simulink model "NPC_grid_tied"  (R2020a)
settings: Solver=ode8  StartTime=0.0  StopTime=0.1  FixedStep=1e-6  RelTol=1e-3
libraries: powerlib x31, simulink x6
(part 2 of 2)

== system NPC_grid_tied/SVPWM/state/2/Subsystem6 ==
  M : Inport
  Constant : Constant  Value=[0 1 0]
  Constant1 : Constant  Value=[1 1 0]
  Constant2 : Constant  Value=[1 1 1]
  Constant3 : Constant  Value=[1 2 1]
  Constant4 : Constant  Value=[1 1 0]
  Constant5 : Constant  Value=[1 1 1]
  Constant6 : Constant  Value=[0 1 0]
  Multiport Switch : MultiPortSwitch  Inputs=7
  state : Outport  VectorParamsAs1DForOutWhenUnconnected=off
  wires:
  Multiport Switch/1 -> state/1
  M/1 -> Multiport Switch/1
  Constant/1 -> Multiport Switch/2
  Constant1/1 -> Multiport Switch/3
  Constant2/1 -> Multiport Switch/4
  Constant3/1 -> Multiport Switch/5
  Constant5/1 -> Multiport Switch/6
  Constant4/1 -> Multiport Switch/7
  Constant6/1 -> Multiport Switch/8

== system NPC_grid_tied/SVPWM/state/2/Subsystem7 ==
  M : Inport
  Constant : Constant  Value=[1 1 0]
  Constant1 : Constant  Value=[1 2 0]
  Constant2 : Constant  Value=[1 2 1]
  Constant3 : Constant  Value=[2 2 1]
  Constant4 : Constant  Value=[1 2 0]
  Constant5 : Constant  Value=[1 2 1]
  Constant6 : Constant  Value=[1 1 0]
  Multiport Switch : MultiPortSwitch  Inputs=7
  state : Outport  VectorParamsAs1DForOutWhenUnconnected=off
  wires:
  Constant6/1 -> Multiport Switch/8
  Constant4/1 -> Multiport Switch/7
  Constant5/1 -> Multiport Switch/6
  Constant3/1 -> Multiport Switch/5
  Constant2/1 -> Multiport Switch/4
  Constant1/1 -> Multiport Switch/3
  Constant/1 -> Multiport Switch/2
  M/1 -> Multiport Switch/1
  Multiport Switch/1 -> state/1

== system NPC_grid_tied/SVPWM/state/2/Subsystem8 ==
  M : Inport
  Constant : Constant  Value=[0 1 0]
  Constant1 : Constant  Value=[1 1 0]
  Constant2 : Constant  Value=[1 2 0]
  Constant3 : Constant  Value=[1 2 1]
  Constant4 : Constant  Value=[1 1 0]
  Constant5 : Constant  Value=[1 2 0]
  Constant6 : Constant  Value=[0 1 0]
  Multiport Switch : MultiPortSwitch  Inputs=7
  state : Outport  VectorParamsAs1DForOutWhenUnconnected=off
  wires:
  Multiport Switch/1 -> state/1
  M/1 -> Multiport Switch/1
  Constant/1 -> Multiport Switch/2
  Constant1/1 -> Multiport Switch/3
  Constant2/1 -> Multiport Switch/4
  Constant3/1 -> Multiport Switch/5
  Constant5/1 -> Multiport Switch/6
  Constant4/1 -> Multiport Switch/7
  Constant6/1 -> Multiport Switch/8

== system NPC_grid_tied/SVPWM/state/2/Subsystem9 ==
  M : Inport
  Constant : Constant  Value=[1 1 0]
  Constant1 : Constant  Value=[1 2 0]
  Constant2 : Constant  Value=[2 2 0]
  Constant3 : Constant  Value=[2 2 1]
  Constant4 : Constant  Value=[1 2 0]
  Constant5 : Constant  Value=[2 2 0]
  Constant6 : Constant  Value=[1 1 0]
  Multiport Switch : MultiPortSwitch  Inputs=7
  state : Outport  VectorParamsAs1DForOutWhenUnconnected=off
  wires:
  Constant6/1 -> Multiport Switch/8
  Constant4/1 -> Multiport Switch/7
  Constant5/1 -> Multiport Switch/6
  Constant3/1 -> Multiport Switch/5
  Constant2/1 -> Multiport Switch/4
  Constant1/1 -> Multiport Switch/3
  Constant/1 -> Multiport Switch/2
  M/1 -> Multiport Switch/1
  Multiport Switch/1 -> state/1

== system NPC_grid_tied/SVPWM/state/3/Subsystem10 ==
  M : Inport
  Constant : Constant  Value=[0 1 1]
  Constant1 : Constant  Value=[0 2 1]
  Constant2 : Constant  Value=[0 2 2]
  Constant3 : Constant  Value=[1 2 2]
  Constant4 : Constant  Value=[0 2 1]
  Constant5 : Constant  Value=[0 2 2]
  Constant6 : Constant  Value=[0 1 1]
  Multiport Switch : MultiPortSwitch  Inputs=7
  state : Outport  VectorParamsAs1DForOutWhenUnconnected=off
  wires:
  Constant6/1 -> Multiport Switch/8
  Constant4/1 -> Multiport Switch/7
  Constant5/1 -> Multiport Switch/6
  Constant3/1 -> Multiport Switch/5
  Constant2/1 -> Multiport Switch/4
  Constant1/1 -> Multiport Switch/3
  Constant/1 -> Multiport Switch/2
  M/1 -> Multiport Switch/1
  Multiport Switch/1 -> state/1

== system NPC_grid_tied/SVPWM/state/3/Subsystem5 ==
  M : Inport
  Constant : Constant  Value=[0 1 0]
  Constant1 : Constant  Value=[0 1 1]
  Constant2 : Constant  Value=[1 1 1]
  Constant3 : Constant  Value=[1 2 1]
  Constant4 : Constant  Value=[0 1 1]
  Constant5 : Constant  Value=[1 1 1]
  Constant6 : Constant  Value=[0 1 0]
  Multiport Switch : MultiPortSwitch  Inputs=7
  state : Outport  VectorParamsAs1DForOutWhenUnconnected=off
  wires:
  Multiport Switch/1 -> state/1
  M/1 -> Multiport Switch/1
  Constant/1 -> Multiport Switch/2
  Constant1/1 -> Multiport Switch/3
  Constant2/1 -> Multiport Switch/4
  Constant3/1 -> Multiport Switch/5
  Constant5/1 -> Multiport Switch/6
  Constant4/1 -> Multiport Switch/7
  Constant6/1 -> Multiport Switch/8

== system NPC_grid_tied/SVPWM/state/3/Subsystem6 ==
  M : Inport
  Constant : Constant  Value=[0 1 1]
  Constant1 : Constant  Value=[1 1 1]
  Constant2 : Constant  Value=[1 2 1]
  Constant3 : Constant  Value=[1 2 2]
  Constant4 : Constant  Value=[1 1 1]
  Constant5 : Constant  Value=[1 2 1]
  Constant6 : Constant  Value=[0 1 1]
  Multiport Switch : MultiPortSwitch  Inputs=7
  state : Outport  VectorParamsAs1DForOutWhenUnconnected=off
  wires:
  Constant6/1 -> Multiport Switch/8
  Constant4/1 -> Multiport Switch/7
  Constant5/1 -> Multiport Switch/6
  Constant3/1 -> Multiport Switch/5
  Constant2/1 -> Multiport Switch/4
  Constant1/1 -> Multiport Switch/3
  Constant/1 -> Multiport Switch/2
  M/1 -> Multiport Switch/1
  Multiport Switch/1 -> state/1

== system NPC_grid_tied/SVPWM/state/3/Subsystem7 ==
  M : Inport
  Constant : Constant  Value=[0 1 0]
  Constant1 : Constant  Value=[0 1 1]
  Constant2 : Constant  Value=[0 2 1]
  Constant3 : Constant  Value=[1 2 1]
  Constant4 : Constant  Value=[0 1 1]
  Constant5 : Constant  Value=[0 2 1]
  Constant6 : Constant  Value=[0 1 0]
  Multiport Switch : MultiPortSwitch  Inputs=7
  state : Outport  VectorParamsAs1DForOutWhenUnconnected=off
  wires:
  Multiport Switch/1 -> state/1
  M/1 -> Multiport Switch/1
  Constant/1 -> Multiport Switch/2
  Constant1/1 -> Multiport Switch/3
  Constant2/1 -> Multiport Switch/4
  Constant3/1 -> Multiport Switch/5
  Constant5/1 -> Multiport Switch/6
  Constant4/1 -> Multiport Switch/7
  Constant6/1 -> Multiport Switch/8

== system NPC_grid_tied/SVPWM/state/3/Subsystem8 ==
  M : Inport
  Constant : Constant  Value=[0 1 1]
  Constant1 : Constant  Value=[0 2 1]
  Constant2 : Constant  Value=[1 2 1]
  Constant3 : Constant  Value=[1 2 2]
  Constant4 : Constant  Value=[0 2 1]
  Constant5 : Constant  Value=[1 2 1]
  Constant6 : Constant  Value=[0 1 1]
  Multiport Switch : MultiPortSwitch  Inputs=7
  state : Outport  VectorParamsAs1DForOutWhenUnconnected=off
  wires:
  Constant6/1 -> Multiport Switch/8
  Constant4/1 -> Multiport Switch/7
  Constant5/1 -> Multiport Switch/6
  Constant3/1 -> Multiport Switch/5
  Constant2/1 -> Multiport Switch/4
  Constant1/1 -> Multiport Switch/3
  Constant/1 -> Multiport Switch/2
  M/1 -> Multiport Switch/1
  Multiport Switch/1 -> state/1

== system NPC_grid_tied/SVPWM/state/3/Subsystem9 ==
  M : Inport
  Constant : Constant  Value=[0 1 0]
  Constant1 : Constant  Value=[0 2 0]
  Constant2 : Constant  Value=[0 2 1]
  Constant3 : Constant  Value=[1 2 1]
  Constant4 : Constant  Value=[0 2 0]
  Constant5 : Constant  Value=[0 2 1]
  Constant6 : Constant  Value=[0 1 0]
  Multiport Switch : MultiPortSwitch  Inputs=7
  state : Outport  VectorParamsAs1DForOutWhenUnconnected=off
  wires:
  Multiport Switch/1 -> state/1
  M/1 -> Multiport Switch/1
  Constant/1 -> Multiport Switch/2
  Constant1/1 -> Multiport Switch/3
  Constant2/1 -> Multiport Switch/4
  Constant3/1 -> Multiport Switch/5
  Constant5/1 -> Multiport Switch/6
  Constant4/1 -> Multiport Switch/7
  Constant6/1 -> Multiport Switch/8

== system NPC_grid_tied/SVPWM/state/4/Subsystem10 ==
  M : Inport
  Constant : Constant  Value=[0 0 1]
  Constant1 : Constant  Value=[0 0 2]
  Constant2 : Constant  Value=[0 1 2]
  Constant3 : Constant  Value=[1 1 2]
  Constant4 : Constant  Value=[0 0 2]
  Constant5 : Constant  Value=[0 1 2]
  Constant6 : Constant  Value=[0 0 1]
  Multiport Switch : MultiPortSwitch  Inputs=7
  state : Outport  VectorParamsAs1DForOutWhenUnconnected=off
  wires:
  Multiport Switch/1 -> state/1
  M/1 -> Multiport Switch/1
  Constant/1 -> Multiport Switch/2
  Constant1/1 -> Multiport Switch/3
  Constant2/1 -> Multiport Switch/4
  Constant3/1 -> Multiport Switch/5
  Constant5/1 -> Multiport Switch/6
  Constant4/1 -> Multiport Switch/7
  Constant6/1 -> Multiport Switch/8

== system NPC_grid_tied/SVPWM/state/4/Subsystem5 ==
  M : Inport
  Constant : Constant  Value=[0 1 1]
  Constant1 : Constant  Value=[1 1 1]
  Constant2 : Constant  Value=[1 1 2]
  Constant3 : Constant  Value=[1 2 2]
  Constant4 : Constant  Value=[1 1 1]
  Constant5 : Constant  Value=[1 1 2]
  Constant6 : Constant  Value=[0 1 1]
  Multiport Switch : MultiPortSwitch  Inputs=7
  state : Outport  VectorParamsAs1DForOutWhenUnconnected=off
  wires:
  Constant6/1 -> Multiport Switch/8
  Constant4/1 -> Multiport Switch/7
  Constant5/1 -> Multiport Switch/6
  Constant3/1 -> Multiport Switch/5
  Constant2/1 -> Multiport Switch/4
  Constant1/1 -> Multiport Switch/3
  Constant/1 -> Multiport Switch/2
  M/1 -> Multiport Switch/1
  Multiport Switch/1 -> state/1

== system NPC_grid_tied/SVPWM/state/4/Subsystem6 ==
  M : Inport
  Constant : Constant  Value=[0 0 1]
  Constant1 : Constant  Value=[0 1 1]
  Constant2 : Constant  Value=[1 1 1]
  Constant3 : Constant  Value=[1 1 2]
  Constant4 : Constant  Value=[0 1 1]
  Constant5 : Constant  Value=[1 1 1]
  Constant6 : Constant  Value=[0 0 1]
  Multiport Switch : MultiPortSwitch  Inputs=7
  state : Outport  VectorParamsAs1DForOutWhenUnconnected=off
  wires:
  Multiport Switch/1 -> state/1
  M/1 -> Multiport Switch/1
  Constant/1 -> Multiport Switch/2
  Constant1/1 -> Multiport Switch/3
  Constant2/1 -> Multiport Switch/4
  Constant3/1 -> Multiport Switch/5
  Constant5/1 -> Multiport Switch/6
  Constant4/1 -> Multiport Switch/7
  Constant6/1 -> Multiport Switch/8

== system NPC_grid_tied/SVPWM/state/4/Subsystem7 ==
  M : Inport
  Constant : Constant  Value=[0 1 1]
  Constant1 : Constant  Value=[0 1 2]
  Constant2 : Constant  Value=[1 1 2]
  Constant3 : Constant  Value=[1 2 2]
  Constant4 : Constant  Value=[0 1 2]
  Constant5 : Constant  Value=[1 1 2]
  Constant6 : Constant  Value=[0 1 1]
  Multiport Switch : MultiPortSwitch  Inputs=7
  state : Outport  VectorParamsAs1DForOutWhenUnconnected=off
  wires:
  Constant6/1 -> Multiport Switch/8
  Constant4/1 -> Multiport Switch/7
  Constant5/1 -> Multiport Switch/6
  Constant3/1 -> Multiport Switch/5
  Constant2/1 -> Multiport Switch/4
  Constant1/1 -> Multiport Switch/3
  Constant/1 -> Multiport Switch/2
  M/1 -> Multiport Switch/1
  Multiport Switch/1 -> state/1

== system NPC_grid_tied/SVPWM/state/4/Subsystem8 ==
  M : Inport
  Constant : Constant  Value=[0 0 1]
  Constant1 : Constant  Value=[0 1 1]
  Constant2 : Constant  Value=[0 1 2]
  Constant3 : Constant  Value=[1 1 2]
  Constant4 : Constant  Value=[0 1 1]
  Constant5 : Constant  Value=[0 1 2]
  Constant6 : Constant  Value=[0 0 1]
  Multiport Switch : MultiPortSwitch  Inputs=7
  state : Outport  VectorParamsAs1DForOutWhenUnconnected=off
  wires:
  Multiport Switch/1 -> state/1
  M/1 -> Multiport Switch/1
  Constant/1 -> Multiport Switch/2
  Constant1/1 -> Multiport Switch/3
  Constant2/1 -> Multiport Switch/4
  Constant3/1 -> Multiport Switch/5
  Constant5/1 -> Multiport Switch/6
  Constant4/1 -> Multiport Switch/7
  Constant6/1 -> Multiport Switch/8

== system NPC_grid_tied/SVPWM/state/4/Subsystem9 ==
  M : Inport
  Constant : Constant  Value=[0 1 1]
  Constant1 : Constant  Value=[0 1 2]
  Constant2 : Constant  Value=[0 2 2]
  Constant3 : Constant  Value=[1 2 2]
  Constant4 : Constant  Value=[0 1 2]
  Constant5 : Constant  Value=[0 2 2]
  Constant6 : Constant  Value=[0 1 1]
  Multiport Switch : MultiPortSwitch  Inputs=7
  state : Outport  VectorParamsAs1DForOutWhenUnconnected=off
  wires:
  Constant6/1 -> Multiport Switch/8
  Constant4/1 -> Multiport Switch/7
  Constant5/1 -> Multiport Switch/6
  Constant3/1 -> Multiport Switch/5
  Constant2/1 -> Multiport Switch/4
  Constant1/1 -> Multiport Switch/3
  Constant/1 -> Multiport Switch/2
  M/1 -> Multiport Switch/1
  Multiport Switch/1 -> state/1

== system NPC_grid_tied/SVPWM/state/5/Subsystem10 ==
  M : Inport
  Constant : Constant  Value=[1 0 1]
  Constant1 : Constant  Value=[1 0 2]
  Constant2 : Constant  Value=[2 0 2]
  Constant3 : Constant  Value=[2 1 2]
  Constant4 : Constant  Value=[1 0 2]
  Constant5 : Constant  Value=[2 0 2]
  Constant6 : Constant  Value=[1 0 1]
  Multiport Switch : MultiPortSwitch  Inputs=7
  state : Outport  VectorParamsAs1DForOutWhenUnconnected=off
  wires:
  Constant6/1 -> Multiport Switch/8
  Constant4/1 -> Multiport Switch/7
  Constant5/1 -> Multiport Switch/6
  Constant3/1 -> Multiport Switch/5
  Constant2/1 -> Multiport Switch/4
  Constant1/1 -> Multiport Switch/3
  Constant/1 -> Multiport Switch/2
  M/1 -> Multiport Switch/1
  Multiport Switch/1 -> state/1

== system NPC_grid_tied/SVPWM/state/5/Subsystem5 ==
  M : Inport
  Constant : Constant  Value=[0 0 1]
  Constant1 : Constant  Value=[1 0 1]
  Constant2 : Constant  Value=[1 1 1]
  Constant3 : Constant  Value=[1 1 2]
  Constant4 : Constant  Value=[1 0 1]
  Constant5 : Constant  Value=[1 1 1]
  Constant6 : Constant  Value=[0 0 1]
  Multiport Switch : MultiPortSwitch  Inputs=7
  state : Outport  VectorParamsAs1DForOutWhenUnconnected=off
  wires:
  Multiport Switch/1 -> state/1
  M/1 -> Multiport Switch/1
  Constant/1 -> Multiport Switch/2
  Constant1/1 -> Multiport Switch/3
  Constant2/1 -> Multiport Switch/4
  Constant3/1 -> Multiport Switch/5
  Constant5/1 -> Multiport Switch/6
  Constant4/1 -> Multiport Switch/7
  Constant6/1 -> Multiport Switch/8

== system NPC_grid_tied/SVPWM/state/5/Subsystem6 ==
  M : Inport
  Constant : Constant  Value=[1 0 1]
  Constant1 : Constant  Value=[1 1 1]
  Constant2 : Constant  Value=[1 1 2]
  Constant3 : Constant  Value=[2 1 2]
  Constant4 : Constant  Value=[1 1 1]
  Constant5 : Constant  Value=[1 1 2]
  Constant6 : Constant  Value=[1 0 1]
  Multiport Switch : MultiPortSwitch  Inputs=7
  state : Outport  VectorParamsAs1DForOutWhenUnconnected=off
  wires:
  Constant6/1 -> Multiport Switch/8
  Constant4/1 -> Multiport Switch/7
  Constant5/1 -> Multiport Switch/6
  Constant3/1 -> Multiport Switch/5
  Constant2/1 -> Multiport Switch/4
  Constant1/1 -> Multiport Switch/3
  Constant/1 -> Multiport Switch/2
  M/1 -> Multiport Switch/1
  Multiport Switch/1 -> state/1

== system NPC_grid_tied/SVPWM/state/5/Subsystem7 ==
  M : Inport
  Constant : Constant  Value=[0 0 1]
  Constant1 : Constant  Value=[1 0 1]
  Constant2 : Constant  Value=[1 0 2]
  Constant3 : Constant  Value=[1 1 2]
  Constant4 : Constant  Value=[1 0 1]
  Constant5 : Constant  Value=[1 0 2]
  Constant6 : Constant  Value=[0 0 1]
  Multiport Switch : MultiPortSwitch  Inputs=7
  state : Outport  VectorParamsAs1DForOutWhenUnconnected=off
  wires:
  Multiport Switch/1 -> state/1
  M/1 -> Multiport Switch/1
  Constant/1 -> Multiport Switch/2
  Constant1/1 -> Multiport Switch/3
  Constant2/1 -> Multiport Switch/4
  Constant3/1 -> Multiport Switch/5
  Constant5/1 -> Multiport Switch/6
  Constant4/1 -> Multiport Switch/7
  Constant6/1 -> Multiport Switch/8

== system NPC_grid_tied/SVPWM/state/5/Subsystem8 ==
  M : Inport
  Constant : Constant  Value=[1 0 1]
  Constant1 : Constant  Value=[1 0 2]
  Constant2 : Constant  Value=[1 1 2]
  Constant3 : Constant  Value=[2 1 2]
  Constant4 : Constant  Value=[1 0 2]
  Constant5 : Constant  Value=[1 1 2]
  Constant6 : Constant  Value=[1 0 1]
  Multiport Switch : MultiPortSwitch  Inputs=7
  state : Outport  VectorParamsAs1DForOutWhenUnconnected=off
  wires:
  Constant6/1 -> Multiport Switch/8
  Constant4/1 -> Multiport Switch/7
  Constant5/1 -> Multiport Switch/6
  Constant3/1 -> Multiport Switch/5
  Constant2/1 -> Multiport Switch/4
  Constant1/1 -> Multiport Switch/3
  Constant/1 -> Multiport Switch/2
  M/1 -> Multiport Switch/1
  Multiport Switch/1 -> state/1

== system NPC_grid_tied/SVPWM/state/5/Subsystem9 ==
  M : Inport
  Constant : Constant  Value=[0 0 1]
  Constant1 : Constant  Value=[0 0 2]
  Constant2 : Constant  Value=[1 0 2]
  Constant3 : Constant  Value=[1 1 2]
  Constant4 : Constant  Value=[0 0 2]
  Constant5 : Constant  Value=[1 0 2]
  Constant6 : Constant  Value=[0 0 1]
  Multiport Switch : MultiPortSwitch  Inputs=7
  state : Outport  VectorParamsAs1DForOutWhenUnconnected=off
  wires:
  Multiport Switch/1 -> state/1
  M/1 -> Multiport Switch/1
  Constant/1 -> Multiport Switch/2
  Constant1/1 -> Multiport Switch/3
  Constant2/1 -> Multiport Switch/4
  Constant3/1 -> Multiport Switch/5
  Constant5/1 -> Multiport Switch/6
  Constant4/1 -> Multiport Switch/7
  Constant6/1 -> Multiport Switch/8

== system NPC_grid_tied/SVPWM/state/6/Subsystem10 ==
  M : Inport
  Constant : Constant  Value=[1 0 0]
  Constant1 : Constant  Value=[2 0 0]
  Constant2 : Constant  Value=[2 0 1]
  Constant3 : Constant  Value=[2 1 1]
  Constant4 : Constant  Value=[2 0 0]
  Constant5 : Constant  Value=[2 0 1]
  Constant6 : Constant  Value=[1 0 0]
  Multiport Switch : MultiPortSwitch  Inputs=7
  state : Outport  VectorParamsAs1DForOutWhenUnconnected=off
  wires:
  Multiport Switch/1 -> state/1
  M/1 -> Multiport Switch/1
  Constant/1 -> Multiport Switch/2
  Constant1/1 -> Multiport Switch/3
  Constant2/1 -> Multiport Switch/4
  Constant3/1 -> Multiport Switch/5
  Constant5/1 -> Multiport Switch/6
  Constant4/1 -> Multiport Switch/7
  Constant6/1 -> Multiport Switch/8

== system NPC_grid_tied/SVPWM/state/6/Subsystem5 ==
  M : Inport
  Constant : Constant  Value=[1 0 1]
  Constant1 : Constant  Value=[1 1 1]
  Constant2 : Constant  Value=[2 1 1]
  Constant3 : Constant  Value=[2 1 2]
  Constant4 : Constant  Value=[1 1 1]
  Constant5 : Constant  Value=[2 1 1]
  Constant6 : Constant  Value=[1 0 1]
  Multiport Switch : MultiPortSwitch  Inputs=7
  state : Outport  VectorParamsAs1DForOutWhenUnconnected=off
  wires:
  Constant6/1 -> Multiport Switch/8
  Constant4/1 -> Multiport Switch/7
  Constant5/1 -> Multiport Switch/6
  Constant3/1 -> Multiport Switch/5
  Constant2/1 -> Multiport Switch/4
  Constant1/1 -> Multiport Switch/3
  Constant/1 -> Multiport Switch/2
  M/1 -> Multiport Switch/1
  Multiport Switch/1 -> state/1

== system NPC_grid_tied/SVPWM/state/6/Subsystem6 ==
  M : Inport
  Constant : Constant  Value=[1 0 0]
  Constant1 : Constant  Value=[1 0 1]
  Constant2 : Constant  Value=[1 1 1]
  Constant3 : Constant  Value=[2 1 1]
  Constant4 : Constant  Value=[1 0 1]
  Constant5 : Constant  Value=[1 1 1]
  Constant6 : Constant  Value=[1 0 0]
  Multiport Switch : MultiPortSwitch  Inputs=7
  state : Outport  VectorParamsAs1DForOutWhenUnconnected=off
  wires:
  Multiport Switch/1 -> state/1
  M/1 -> Multiport Switch/1
  Constant/1 -> Multiport Switch/2
  Constant1/1 -> Multiport Switch/3
  Constant2/1 -> Multiport Switch/4
  Constant3/1 -> Multiport Switch/5
  Constant5/1 -> Multiport Switch/6
  Constant4/1 -> Multiport Switch/7
  Constant6/1 -> Multiport Switch/8

== system NPC_grid_tied/SVPWM/state/6/Subsystem7 ==
  M : Inport
  Constant : Constant  Value=[1 0 1]
  Constant1 : Constant  Value=[2 0 1]
  Constant2 : Constant  Value=[2 1 1]
  Constant3 : Constant  Value=[2 1 2]
  Constant4 : Constant  Value=[2 0 1]
  Constant5 : Constant  Value=[2 1 1]
  Constant6 : Constant  Value=[1 0 1]
  Multiport Switch : MultiPortSwitch  Inputs=7
  state : Outport  VectorParamsAs1DForOutWhenUnconnected=off
  wires:
  Constant6/1 -> Multiport Switch/8
  Constant4/1 -> Multiport Switch/7
  Constant5/1 -> Multiport Switch/6
  Constant3/1 -> Multiport Switch/5
  Constant2/1 -> Multiport Switch/4
  Constant1/1 -> Multiport Switch/3
  Constant/1 -> Multiport Switch/2
  M/1 -> Multiport Switch/1
  Multiport Switch/1 -> state/1

== system NPC_grid_tied/SVPWM/state/6/Subsystem8 ==
  M : Inport
  Constant : Constant  Value=[1 0 0]
  Constant1 : Constant  Value=[1 0 1]
  Constant2 : Constant  Value=[2 0 1]
  Constant3 : Constant  Value=[2 1 1]
  Constant4 : Constant  Value=[1 0 1]
  Constant5 : Constant  Value=[2 0 1]
  Constant6 : Constant  Value=[1 0 0]
  Multiport Switch : MultiPortSwitch  Inputs=7
  state : Outport  VectorParamsAs1DForOutWhenUnconnected=off
  wires:
  Multiport Switch/1 -> state/1
  M/1 -> Multiport Switch/1
  Constant/1 -> Multiport Switch/2
  Constant1/1 -> Multiport Switch/3
  Constant2/1 -> Multiport Switch/4
  Constant3/1 -> Multiport Switch/5
  Constant5/1 -> Multiport Switch/6
  Constant4/1 -> Multiport Switch/7
  Constant6/1 -> Multiport Switch/8

== system NPC_grid_tied/SVPWM/state/6/Subsystem9 ==
  M : Inport
  Constant : Constant  Value=[1 0 1]
  Constant1 : Constant  Value=[2 0 1]
  Constant2 : Constant  Value=[2 0 2]
  Constant3 : Constant  Value=[2 1 2]
  Constant4 : Constant  Value=[2 0 1]
  Constant5 : Constant  Value=[2 0 2]
  Constant6 : Constant  Value=[1 0 1]
  Multiport Switch : MultiPortSwitch  Inputs=7
  state : Outport  VectorParamsAs1DForOutWhenUnconnected=off
  wires:
  Constant6/1 -> Multiport Switch/8
  Constant4/1 -> Multiport Switch/7
  Constant5/1 -> Multiport Switch/6
  Constant3/1 -> Multiport Switch/5
  Constant2/1 -> Multiport Switch/4
  Constant1/1 -> Multiport Switch/3
  Constant/1 -> Multiport Switch/2
  M/1 -> Multiport Switch/1
  Multiport Switch/1 -> state/1

== matlab function NPC_grid_tied/SVPWM/T ==
  data: theta input; T01 output; T02 output; m input; Ts input; T2 output; T3 output; N input; n input; k input; Ia input; Ib input; Ic input
function [T01,T02,T2,T3] = fcn(theta,m,Ts,N,n,k,Ia,Ib,Ic)

if N == 1
    switch (n)
        case 1
            T2 = 2*m*Ts*sin(theta);
            T3 = Ts*(1-2*m*sin(pi/3+theta));
        case 2
            T2 = Ts*(1-2*m*sin(pi/3+theta));
            T3 = 2*m*Ts*sin(pi/3-theta);
        case 3
            T2 = Ts*(1-2*m*sin(pi/3-theta));
            T3 = Ts*(2*m*sin(pi/3+theta)-1);
        case 4
            T2 = Ts*(2*m*sin(pi/3+theta)-1);
            T3 = Ts*(1-2*m*sin(theta));
        case 5
            T2 = Ts*(2*m*sin(pi/3-theta)-1);
            T3 = 2*m*Ts*sin(theta);
        case 6
            T2 = 2*m*Ts*sin(pi/3-theta);
            T3 = Ts*(2*m*sin(theta)-1);
        otherwise
            %Should never reach this
            T01 = 0;
            T02 = 0;
            T2 = 0;
            T3 = 0;
    end
    
    if(n == 1 || n == 3 || n == 5)
         if(Ia>0)
        %add to handle Over modulation
        if (T2 + T3 > Ts)
            T2 = T2 * Ts /(T2 + T3);
            T3 = T3 * Ts /(T2 + T3);
            T01 = 0;
            T02 = 0;
        else
         %add to handle Bus Balance
            T2 = T2;
            T3 = T3;
            %T1 = Ts - T2 - T3;
            T01 = (k + 0.5)*(Ts - T2 - T3);
            T02 = (Ts - T2 - T3) - T01;
        end
    else
         if (T2 + T3 > Ts)
            T2 = T2 * Ts /(T2 + T3);
            T3 = T3 * Ts /(T2 + T3);
            T01 = 0;
            T02 = 0;
        else
            T2 = T2;
            T3 = T3;
            %T1 = Ts - T2 - T3;
            T02 = (k + 0.5)*(Ts - T2 - T3);
            T01 = (Ts - T2 - T3) - T02;
        end
    end
    else
         if((-Ic)>0)
            %add to handle Over modulation
            if (T2 + T3 > Ts)
                T2 = T2 * Ts /(T2 + T3);
                T3 = T3 * Ts /(T2 + T3);
                T01 = 0;
                T02 = 0;
            else
             %add to handle Bus Balance
                T2 = T2;
                T3 = T3;
                %T1 = Ts - T2 - T3;
                T01 = (k + 0.5)*(Ts - T2 - T3);
                T02 = (Ts - T2 - T3) - T01;
            end
       else
         if (T2 + T3 > Ts)
            T2 = T2 * Ts /(T2 + T3);
            T3 = T3 * Ts /(T2 + T3);
            T01 = 0;
            T02 = 0;
           else
            T2 = T2;
            T3 = T3;
            %T1 = Ts - T2 - T3;
            T02 = (k + 0.5)*(Ts - T2 - T3);
            T01 = (Ts - T2 - T3) - T02;
         end
      end
    end
elseif N == 2
    switch (n)
         case 1
            T2 = Ts*(1-2*m*sin(pi/3+theta));
            T3 = 2*m*Ts*sin(theta);
        case 2
            T2 = 2*m*Ts*sin(pi/3-theta);
            T3 = Ts*(1-2*m*sin(pi/3+theta));
        case 3
            T2 = Ts*(2*m*sin(pi/3+theta)-1);
            T3 = Ts*(1-2*m*sin(pi/3-theta));
        case 4
            T2 = Ts*(1-2*m*sin(theta));
            T3 = Ts*(2*m*sin(pi/3+theta)-1);
        case 5
            T2 = 2*m*Ts*sin(theta);
            T3 = Ts*(2*m*sin(pi/3-theta)-1);
        case 6
            T2 = Ts*(2*m*sin(theta)-1);
            T3 = 2*m*Ts*sin(pi/3-theta);
        otherwise
            T01 = 0;
            T02 = 0;
            T2 = 0;
            T3 = 0;
    end
    
        if(n == 1 || n == 3 || n == 5)
         if((-Ic)>0)
        %add to handle Over modulation
        if (T2 + T3 > Ts)
            T2 = T2 * Ts /(T2 + T3);
            T3 = T3 * Ts /(T2 + T3);
            T01 = 0;
            T02 = 0;
        else
         %add to handle Bus Balance
            T2 = T2;
            T3 = T3;
            %T1 = Ts - T2 - T3;
            T01 = (k + 0.5)*(Ts - T2 - T3);
            T02 = (Ts - T2 - T3) - T01;
        end
    else
         if (T2 + T3 > Ts)
            T2 = T2 * Ts /(T2 + T3);
            T3 = T3 * Ts /(T2 + T3);
            T01 = 0;
            T02 = 0;
        else
            T2 = T2;
            T3 = T3;
            %T1 = Ts - T2 - T3;
            T02 = (k + 0.5)*(Ts - T2 - T3);
            T01 = (Ts - T2 - T3) - T02;
        end
    end
    else
         if((Ib)>0)
            %add to handle Over modulation
            if (T2 + T3 > Ts)
                T2 = T2 * Ts /(T2 + T3);
                T3 = T3 * Ts /(T2 + T3);
                T01 = 0;
                T02 = 0;
            else
             %add to handle Bus Balance
                T2 = T2;
                T3 = T3;
                %T1 = Ts - T2 - T3;
                T01 = (k + 0.5)*(Ts - T2 - T3);
                T02 = (Ts - T2 - T3) - T01;
            end
       else
         if (T2 + T3 > Ts)
            T2 = T2 * Ts /(T2 + T3);
            T3 = T3 * Ts /(T2 + T3);
            T01 = 0;
            T02 = 0;
           else
            T2 = T2;
            T3 = T3;
            %T1 = Ts - T2 - T3;
            T02 = (k + 0.5)*(Ts - T2 - T3);
            T01 = (Ts - T2 - T3) - T02;
         end
      end
    end
    
elseif N == 3
    switch (n)
         case 1
            T2 = 2*m*Ts*sin(theta);
            T3 = Ts*(1-2*m*sin(pi/3+theta));
        case 2
            T2 = Ts*(1-2*m*sin(pi/3+theta));
            T3 = 2*m*Ts*sin(pi/3-theta);
        case 3
            T2 = Ts*(1-2*m*sin(pi/3-theta));
            T3 = Ts*(2*m*sin(pi/3+theta)-1);
        case 4
            T2 = Ts*(2*m*sin(pi/3+theta)-1);
            T3 = Ts*(1-2*m*sin(theta));
        case 5
            T2 = Ts*(2*m*sin(pi/3-theta)-1);
            T3 = 2*m*Ts*sin(theta);
        case 6
            T2 = 2*m*Ts*sin(pi/3-theta);
            T3 = Ts*(2*m*sin(theta)-1);
        otherwise
            T01 = 0;
            T02 = 0;
            T2 = 0;
            T3 = 0;
    end
    
        if(n == 1 || n == 3 || n == 5)
         if(Ib>0)
        %add to handle Over modulation
        if (T2 + T3 > Ts)
            T2 = T2 * Ts /(T2 + T3);
            T3 = T3 * Ts /(T2 + T3);
            T01 = 0;
            T02 = 0;
        else
         %add to handle Bus Balance
            T2 = T2;
            T3 = T3;
            %T1 = Ts - T2 - T3;
            T01 = (k + 0.5)*(Ts - T2 - T3);
            T02 = (Ts - T2 - T3) - T01;
        end
    else
         if (T2 + T3 > Ts)
            T2 = T2 * Ts /(T2 + T3);
            T3 = T3 * Ts /(T2 + T3);
            T01 = 0;
            T02 = 0;
        else
            T2 = T2;
            T3 = T3;
            %T1 = Ts - T2 - T3;
            T02 = (k + 0.5)*(Ts - T2 - T3);
            T01 = (Ts - T2 - T3) - T02;
        end
    end
    else
         if((-Ia)>0)
            %add to handle Over modulation
            if (T2 + T3 > Ts)
                T2 = T2 * Ts /(T2 + T3);
                T3 = T3 * Ts /(T2 + T3);
                T01 = 0;
                T02 = 0;
            else
             %add to handle Bus Balance
                T2 = T2;
                T3 = T3;
                %T1 = Ts - T2 - T3;
                T01 = (k + 0.5)*(Ts - T2 - T3);
                T02 = (Ts - T2 - T3) - T01;
            end
       else
         if (T2 + T3 > Ts)
            T2 = T2 * Ts /(T2 + T3);
            T3 = T3 * Ts /(T2 + T3);
            T01 = 0;
            T02 = 0;
           else
            T2 = T2;
            T3 = T3;
            %T1 = Ts - T2 - T3;
            T02 = (k + 0.5)*(Ts - T2 - T3);
            T01 = (Ts - T2 - T3) - T02;
         end
      end
    end
elseif N == 4
    switch (n)
         case 1
            T2 = Ts*(1-2*m*sin(pi/3+theta));
            T3 = 2*m*Ts*sin(theta);
        case 2
            T2 = 2*m*Ts*sin(pi/3-theta);
            T3 = Ts*(1-2*m*sin(pi/3+theta));
        case 3
            T2 = Ts*(2*m*sin(pi/3+theta)-1);
            T3 = Ts*(1-2*m*sin(pi/3-theta));
        case 4
            T2 = Ts*(1-2*m*sin(theta));
            T3 = Ts*(2*m*sin(pi/3+theta)-1);
        case 5
            T2 = 2*m*Ts*sin(theta);
            T3 = Ts*(2*m*sin(pi/3-theta)-1);
        case 6
            T2 = Ts*(2*m*sin(theta)-1);
            T3 = 2*m*Ts*sin(pi/3-theta);
        otherwise
           T01 = 0;
           T02 = 0;
           T2 = 0;
           T3 = 0;
    end
    
       if(n == 1 || n == 3 || n == 5)
         if((-Ia)>0)
        %add to handle Over modulation
        if (T2 + T3 > Ts)
            T2 = T2 * Ts /(T2 + T3);
            T3 = T3 * Ts /(T2 + T3);
            T01 = 0;
            T02 = 0;
        else
         %add to handle Bus Balance
            T2 = T2;
            T3 = T3;
            %T1 = Ts - T2 - T3;
            T01 = (k + 0.5)*(Ts - T2 - T3);
            T02 = (Ts - T2 - T3) - T01;
        end
    else
         if (T2 + T3 > Ts)
            T2 = T2 * Ts /(T2 + T3);
            T3 = T3 * Ts /(T2 + T3);
            T01 = 0;
            T02 = 0;
        else
            T2 = T2;
            T3 = T3;
            %T1 = Ts - T2 - T3;
            T02 = (k + 0.5)*(Ts - T2 - T3);
            T01 = (Ts - T2 - T3) - T02;
        end
    end
    else
         if(Ic>0)
            %add to handle Over modulation
            if (T2 + T3 > Ts)
                T2 = T2 * Ts /(T2 + T3);
                T3 = T3 * Ts /(T2 + T3);
                T01 = 0;
                T02 = 0;
            else
             %add to handle Bus Balance
                T2 = T2;
                T3 = T3;
                %T1 = Ts - T2 - T3;
                T01 = (k + 0.5)*(Ts - T2 - T3);
                T02 = (Ts - T2 - T3) - T01;
            end
       else
         if (T2 + T3 > Ts)
            T2 = T2 * Ts /(T2 + T3);
            T3 = T3 * Ts /(T2 + T3);
            T01 = 0;
            T02 = 0;
           else
            T2 = T2;
            T3 = T3;
            %T1 = Ts - T2 - T3;
            T02 = (k + 0.5)*(Ts - T2 - T3);
            T01 = (Ts - T2 - T3) - T02;
         end
      end
    end
elseif N == 5
    switch (n)
         case 1
            T2 = 2*m*Ts*sin(theta);
            T3 = Ts*(1-2*m*sin(pi/3+theta));
        case 2
            T2 = Ts*(1-2*m*sin(pi/3+theta));
            T3 = 2*m*Ts*sin(pi/3-theta);
        case 3
            T2 = Ts*(1-2*m*sin(pi/3-theta));
            T3 = Ts*(2*m*sin(pi/3+theta)-1);
        case 4
            T2 = Ts*(2*m*sin(pi/3+theta)-1);
            T3 = Ts*(1-2*m*sin(theta));
        case 5
            T2 = Ts*(2*m*sin(pi/3-theta)-1);
            T3 = 2*m*Ts*sin(theta);
        case 6
            T2 = 2*m*Ts*sin(pi/3-theta);
            T3 = Ts*(2*m*sin(theta)-1);
        otherwise
           T01 = 0;
           T02 = 0;
           T2 = 0;
           T3 = 0;
    end
    
     if(n == 1 || n == 3 || n == 5)
         if((Ic)>0)
        %add to handle Over modulation
        if (T2 + T3 > Ts)
            T2 = T2 * Ts /(T2 + T3);
            T3 = T3 * Ts /(T2 + T3);
            T01 = 0;
            T02 = 0;
        else
         %add to handle Bus Balance
            T2 = T2;
            T3 = T3;
            %T1 = Ts - T2 - T3;
            T01 = (k + 0.5)*(Ts - T2 - T3);
            T02 = (Ts - T2 - T3) - T01;
        end
    else
         if (T2 + T3 > Ts)
            T2 = T2 * Ts /(T2 + T3);
            T3 = T3 * Ts /(T2 + T3);
            T01 = 0;
            T02 = 0;
        else
            T2 = T2;
            T3 = T3;
            %T1 = Ts - T2 - T3;
            T02 = (k + 0.5)*(Ts - T2 - T3);
            T01 = (Ts - T2 - T3) - T02;
        end
    end
    else
         if((-Ib)>0)
            %add to handle Over modulation
            if (T2 + T3 > Ts)
                T2 = T2 * Ts /(T2 + T3);
                T3 = T3 * Ts /(T2 + T3);
                T01 = 0;
                T02 = 0;
            else
             %add to handle Bus Balance
                T2 = T2;
                T3 = T3;
                %T1 = Ts - T2 - T3;
                T01 = (k + 0.5)*(Ts - T2 - T3);
                T02 = (Ts - T2 - T3) - T01;
            end
       else
         if (T2 + T3 > Ts)
            T2 = T2 * Ts /(T2 + T3);
            T3 = T3 * Ts /(T2 + T3);
            T01 = 0;
            T02 = 0;
           else
            T2 = T2;
            T3 = T3;
            %T1 = Ts - T2 - T3;
            T02 = (k + 0.5)*(Ts - T2 - T3);
            T01 = (Ts - T2 - T3) - T02;
         end
      end
    end
elseif N == 6
    switch (n)
         case 1
            T2 = Ts*(1-2*m*sin(pi/3+theta));
            T3 = 2*m*Ts*sin(theta);
        case 2
            T2 = 2*m*Ts*sin(pi/3-theta);
            T3 = Ts*(1-2*m*sin(pi/3+theta));
        case 3
            T2 = Ts*(2*m*sin(pi/3+theta)-1);
            T3 = Ts*(1-2*m*sin(pi/3-theta));
        case 4
            T2 = Ts*(1-2*m*sin(theta));
            T3 = Ts*(2*m*sin(pi/3+theta)-1);
        case 5
            T2 = 2*m*Ts*sin(theta);
            T3 = Ts*(2*m*sin(pi/3-theta)-1);
        case 6
            T2 = Ts*(2*m*sin(theta)-1);
            T3 = 2*m*Ts*sin(pi/3-theta);
        otherwise
            T01 = 0;
            T02 = 0;
            T2 = 0;
            T3 = 0;
    end
    
   if(n == 1 || n == 3 || n == 5)
         if((-Ib)>0)
        %add to handle Over modulation
        if (T2 + T3 > Ts)
            T2 = T2 * Ts /(T2 + T3);
            T3 = T3 * Ts /(T2 + T3);
            T01 = 0;
            T02 = 0;
        else
         %add to handle Bus Balance
            T2 = T2;
            T3 = T3;
            %T1 = Ts - T2 - T3;
            T01 = (k + 0.5)*(Ts - T2 - T3);
            T02 = (Ts - T2 - T3) - T01;
        end
    else
         if (T2 + T3 > Ts)
            T2 = T2 * Ts /(T2 + T3);
            T3 = T3 * Ts /(T2 + T3);
            T01 = 0;
            T02 = 0;
        else
            T2 = T2;
            T3 = T3;
            %T1 = Ts - T2 - T3;
            T02 = (k + 0.5)*(Ts - T2 - T3);
            T01 = (Ts - T2 - T3) - T02;
        end
    end
    else
         if(Ia>0)
            %add to handle Over modulation
            if (T2 + T3 > Ts)
                T2 = T2 * Ts /(T2 + T3);
                T3 = T3 * Ts /(T2 + T3);
                T01 = 0;
                T02 = 0;
            else
             %add to handle Bus Balance
                T2 = T2;
                T3 = T3;
                %T1 = Ts - T2 - T3;
                T01 = (k + 0.5)*(Ts - T2 - T3);
                T02 = (Ts - T2 - T3) - T01;
            end
       else
         if (T2 + T3 > Ts)
            T2 = T2 * Ts /(T2 + T3);
            T3 = T3 * Ts /(T2 + T3);
            T01 = 0;
            T02 = 0;
           else
            T2 = T2;
            T3 = T3;
            %T1 = Ts - T2 - T3;
            T02 = (k + 0.5)*(Ts - T2 - T3);
            T01 = (Ts - T2 - T3) - T02;
         end
      end
    end
else
  T01 = 0;
  T02 = 0;
  T2 = 0;
  T3 = 0;
end
